simulink model "Three_Phase_Bridge_All_controlled"  (Simulink 7.5)
settings: Solver=ode15s  StartTime=0.0  StopTime=0.1  RelTol=1e-3
undefined symbols (not defined in the file): D11, Delta
libraries: powerlib x17, powerlib_extras x3
settings Model: Creator=lm  LastModifiedBy=lm

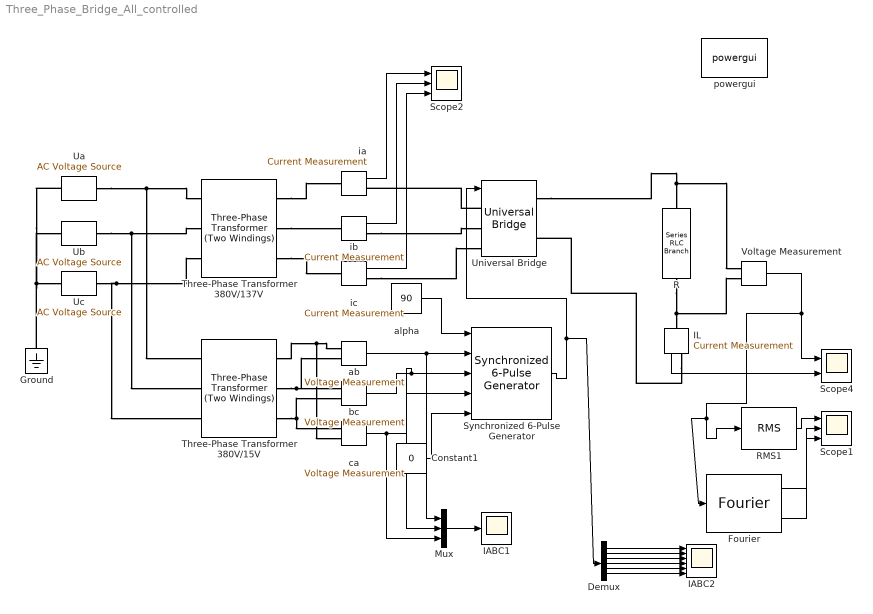
== system Three_Phase_Bridge_All_controlled ==
  Constant1 : Constant  Value=0  OutDataType=fixdt(1, 16)  OutScaling=2^0
  Demux : Demux  Outputs=6
  Fourier : powerlib_extras/Measurements/Fourier  DialogController=POWERSYS.PowerSysDialog  SystemSampleTime=-1  f1=50  n=6
  Ground : powerlib/Elements/Ground  DialogController=POWERSYS.PowerSysDialog  PhysicalDomain=powersysdomain  SubClassName=unknown  LeftPortType=p1  RightPortType=p1  LConnTagsString=a
  IABC1 : Scope
      settings: TimeRange=0.1  YMin=-30  YMax=30
  IABC2 : Scope  NumInputPorts=6
      settings: YMin=-0.003~-129.8~129.75~-5~-5~-5  YMax=0.003~-129.75~129.8~5~5~5  SaveName=ScopeData3
  IL : powerlib/Measurements/Current Measurement  DialogController=POWERSYS.PowerSysDialog  SystemSampleTime=-1  PhasorSimulation=off  OutputType=Complex  PSBequivalent=0
  Mux : Mux  Inputs=3
  R : powerlib/Elements/Series RLC Branch  DialogController=POWERSYS.PowerSysDialog  PhysicalDomain=powersysdomain  SubClassName=unknown  LeftPortType=p1  RightPortType=p1  LConnTagsString=__new0  RConnTagsString=__new0  BranchType=RL  Resistance=5  Inductance=1e-2  SetiL0=off  InitialCurrent=0  Capacitance=1e-6  Setx0=off  InitialVoltage=0  Measurements=None
  RMS1 : powerlib_extras/Measurements/RMS  DialogController=POWERSYS.PowerSysDialog  SystemSampleTime=-1  f1=60
  Scope1 : Scope  NumInputPorts=3
      settings: TimeRange=0.1  YMin=0~0~-5  YMax=1000~500~5
  Scope2 : Scope  NumInputPorts=3
      settings: TimeRange=0.1  YMin=0~0~-5  YMax=1000~500~5  SaveName=ScopeData2
  Scope4 : Scope  NumInputPorts=2
      settings: TimeRange=0.1  YMin=0~0  YMax=1000~500  SaveName=ScopeData4
  Synchronized 6-Pulse Generator : powerlib_extras/Control  Blocks/Synchronized 6-Pulse Generator  DialogController=POWERSYS.PowerSysDialog  SystemSampleTime=-1  freq=50  pwidth=1  Double_Pulse=on
  Three-Phase Transformer 380V/137V : powerlib/Elements/Three-Phase Transformer (Two Windings)  DialogController=POWERSYS.PowerSysDialog  SystemSampleTime=-1  Winding1Connection=Delta (D11)  UNITS=SI  NominalPower=[ 250e6 , 50 ]  Winding1=[380 3.4656e-006 4.4125e-007]  Winding2Connection=Y  Winding2=[173 2.3943e-007 3.0485e-008]  SetSaturation=off  Rm=0.8664  Lm=0.0027578  Saturation=[0 0;744.32 2.0527;3.1013e+005 2.6001]  Hysteresis=off  DataFile='hysteresis'  SetInitialFlux=off  InitialFluxes=[1.3685 -1.3685 1.1974]  Measurements=Winding voltages  MoreParameters=off  BreakLoop=off  DataType=on  TransfoNumber=1
  Three-Phase Transformer 380V/15V : powerlib/Elements/Three-Phase Transformer (Two Windings)  DialogController=POWERSYS.PowerSysDialog  SystemSampleTime=-1  Winding1Connection=Delta (D11)  UNITS=pu  NominalPower=[ 250e6 , 50 ]  Winding1=[380 0.0013407 0.053629]  Winding2Connection=Y  Winding2=[15 0.26603 10.641]  SetSaturation=off  Rm=335.18  Lm=335.17  Saturation=[0 0;0.0029312 0.98252;1.2213 1.2445]  Hysteresis=off  DataFile='hysteresis'  SetInitialFlux=off  InitialFluxes=[0.65503 -0.65503 0.57313]  Measurements=None  MoreParameters=off  BreakLoop=off  DataType=off  TransfoNumber=1
  Ua : powerlib/Electrical Sources/AC Voltage Source  DialogController=POWERSYS.PowerSysDialog  SystemSampleTime=-1  Amplitude=380  Phase=0  Frequency=50  SampleTime=0  Measurements=None
  Ub : powerlib/Electrical Sources/AC Voltage Source  DialogController=POWERSYS.PowerSysDialog  SystemSampleTime=-1  Amplitude=380  Phase=-120  Frequency=50  SampleTime=0  Measurements=None
  Uc : powerlib/Electrical Sources/AC Voltage Source  DialogController=POWERSYS.PowerSysDialog  SystemSampleTime=-1  Amplitude=380  Phase=-240  Frequency=50  SampleTime=0  Measurements=None
  Universal Bridge : powerlib/Power Electronics/Universal Bridge  DialogController=POWERSYS.PowerSysDialog  SystemSampleTime=-1  Arms=3  SnubberResistance=1e5  SnubberCapacitance=inf  Device=Thyristors  Ron=1e-3  Lon=0  ForwardVoltages="[  0  0  ]"  ForwardVoltage=0  GTOparameters=[ 10e-6 , 20e-6 ]  IGBTparameters=[ 1e-6 , 2e-6 ]  Measurements=None  Measurements_2=None  converterType=Rectifier
  Voltage Measurement : powerlib/Measurements/Voltage Measurement  DialogController=POWERSYS.PowerSysDialog  SystemSampleTime=-1  PhasorSimulation=off  OutputType=Complex  PSBequivalent=0
  ab : powerlib/Measurements/Voltage Measurement  DialogController=POWERSYS.PowerSysDialog  SystemSampleTime=-1  PhasorSimulation=off  OutputType=Complex  PSBequivalent=0
  alpha : Constant  Value=90  OutDataType=fixdt(1, 16)  OutScaling=2^0
  bc : powerlib/Measurements/Voltage Measurement  DialogController=POWERSYS.PowerSysDialog  SystemSampleTime=-1  PhasorSimulation=off  OutputType=Complex  PSBequivalent=0
  ca : powerlib/Measurements/Voltage Measurement  DialogController=POWERSYS.PowerSysDialog  SystemSampleTime=-1  PhasorSimulation=off  OutputType=Complex  PSBequivalent=0
  ia : powerlib/Measurements/Current Measurement  DialogController=POWERSYS.PowerSysDialog  SystemSampleTime=-1  PhasorSimulation=off  OutputType=Complex  PSBequivalent=0
  ib : powerlib/Measurements/Current Measurement  DialogController=POWERSYS.PowerSysDialog  SystemSampleTime=-1  PhasorSimulation=off  OutputType=Complex  PSBequivalent=0
  ic : powerlib/Measurements/Current Measurement  DialogController=POWERSYS.PowerSysDialog  SystemSampleTime=-1  PhasorSimulation=off  OutputType=Complex  PSBequivalent=0
  powergui : powerlib/powergui  Priority=1  SystemSampleTime=-1  SimulationMode=Discrete  SampleTime=50e-6  frequency=60  SPID=off  DisableSnubberDevices=off  DisableRonSwitches=off  DisableVfSwitches=off  SwTol=0  Interpol=off  frequencyindice=50  echomessages=off  HookPort=off  DisplayEquations=off  FunctionMessages=off  EnableUseOfTLC=off  x0status=blocks  RestoreLinks=warning  ResistiveCurrentMeasurement=off  Ylog=off  Xlog=on  ShowGrid=off  save=off  variable=ZData  ZoomFFT=off  StartTime=0.0  cycles=1  DisplayStyle=1  FreqAxis=off  MaxFrequency=1000  frequencyindicesteady=1  display=off  methode=off
  wires:
  ab/1 -> Synchronized 6-Pulse Generator/2, Mux/1
  bc/1 -> Synchronized 6-Pulse Generator/3, Mux/2
  ca/1 -> Synchronized 6-Pulse Generator/4, Mux/3
  Synchronized 6-Pulse Generator/1 -> Universal Bridge/1, Demux/1
  Voltage Measurement/1 -> Scope4/1, RMS1/1, Fourier/1
  IL/1 -> Scope4/2
  alpha/1 -> Synchronized 6-Pulse Generator/1
  Constant1/1 -> Synchronized 6-Pulse Generator/5
  Demux/1 -> IABC2/1
  Demux/2 -> IABC2/2
  Demux/3 -> IABC2/3
  Demux/4 -> IABC2/4
  Demux/5 -> IABC2/5
  Demux/6 -> IABC2/6
  Mux/1 -> IABC1/1
  RMS1/1 -> Scope1/1
  Fourier/1 -> Scope1/2
  Fourier/2 -> Scope1/3
  ia/1 -> Scope2/1
  ib/1 -> Scope2/2
  ic/1 -> Scope2/3
  connections:
  R/LConn1 -- IL/LConn1 -- Voltage Measurement/LConn2
  Ground/LConn1 -- Ua/LConn1 -- Ub/LConn1 -- Uc/LConn1
  Ua/RConn1 -- Three-Phase Transformer 380V/137V/LConn1 -- Three-Phase Transformer 380V/15V/LConn1
  Ub/RConn1 -- Three-Phase Transformer 380V/137V/LConn2 -- Three-Phase Transformer 380V/15V/LConn2
  Uc/RConn1 -- Three-Phase Transformer 380V/137V/LConn3 -- Three-Phase Transformer 380V/15V/LConn3
  Universal Bridge/RConn1 -- R/RConn1 -- Voltage Measurement/LConn1
  IL/RConn1 -- Universal Bridge/RConn2
  Three-Phase Transformer 380V/15V/RConn1 -- ab/LConn1 -- ca/LConn2
  Three-Phase Transformer 380V/15V/RConn2 -- ab/LConn2 -- bc/LConn1
  Three-Phase Transformer 380V/15V/RConn3 -- bc/LConn2 -- ca/LConn1
  Three-Phase Transformer 380V/137V/RConn1 -- ia/LConn1
  Universal Bridge/LConn1 -- ia/RConn1
  Three-Phase Transformer 380V/137V/RConn2 -- ib/LConn1
  ib/RConn1 -- Universal Bridge/LConn2
  Three-Phase Transformer 380V/137V/RConn3 -- ic/LConn1
  ic/RConn1 -- Universal Bridge/LConn3
